simulink model "nl_cart_3"  (R2022a)
settings: Solver=ode45  StartTime=0.0  StopTime=40  MaxStep=0.001  MinStep=0.000001  RelTol=1e-3
values from neighbouring files (symbols this model uses):
  b = 0    [ex1.m]    (also in ex2.m = 1; ex3.m = 1; lab3es2_20230414.m = 1)
  dth0 = 0    [ex1.m]    (also in ex2.m; ex3.m)
  dx0 = 0    [ex1.m]    (also in ex2.m; ex3.m)
  g = 9.81    [ex1.m]    (also in ex2.m; ex3.m; lab3es2_20230414.m)
  Ie = I + m * l^2    (= 0.02603525)    [ex1.m]    (also in ex2.m; ex3.m; lab3es2_20230414.m = 0.026047)
  K = [k1, k2, k3, k4]    [ex3.m]    (also in lab3es2_20230414.m = [k,0,0,0])
  l = 0.305    [ex1.m]    (also in ex2.m; ex3.m; lab3es2_20230414.m)
  m = 0.21    [ex1.m]    (also in ex2.m; ex3.m; lab3es2_20230414.m)
  Me = M + m    (= 0.665)    [ex1.m]    (also in ex2.m; ex3.m; lab3es2_20230414.m)
  th0 = pi    (= 3.14159265359)    [ex1.m]    (also in ex2.m = 0; ex3.m = 0)
  x0 = 0    [ex1.m]    (also in ex2.m; ex3.m = 10)
undefined symbols (not defined in the file or in its folder): d
settings Model: Creator=loren  LastModifiedBy=loren
settings DataIOCC: ReturnWorkspaceOutputs=off

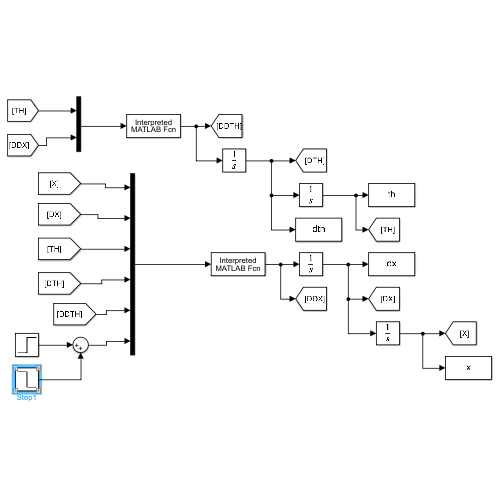
[thumbnail: Simulink's stored preview of the top-level diagram]
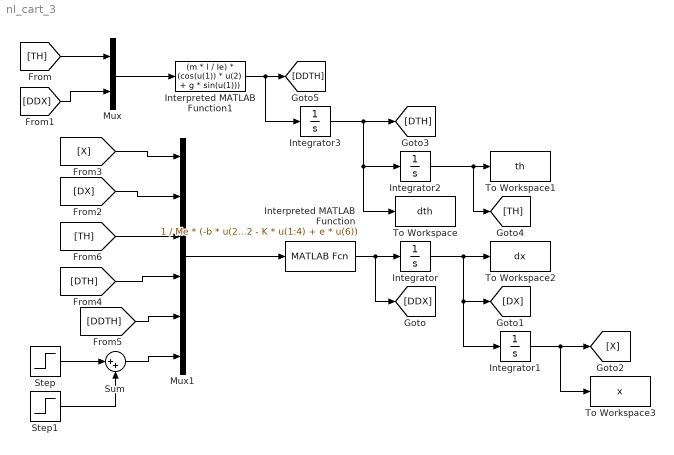
== system nl_cart_3 ==
  Integrator : Integrator  InitialCondition=dx0
  Integrator1 : Integrator  InitialCondition=x0
  Integrator2 : Integrator  InitialCondition=th0
  Integrator3 : Integrator  InitialCondition=dth0
  Interpreted MATLAB Function : MATLABFcn  MATLABFcn=1 / Me * (-b * u(2) + m * l * cos(u(3)) * u(5) - m * l * sin(u(3)) * u(4)^2 - K * u(1:4) + e * u(6))  OutputDimensions=1
  Interpreted MATLAB Function1 : MATLABFcn  MATLABFcn=(m * l / Ie) * (cos(u(1)) * u(2) + g * sin(u(1)))  OutputDimensions=1
  Mux : Mux  Inputs=2
  Mux1 : Mux  Inputs=6
  Step : Step  Time=d.start  After=d.A  SampleTime=0
  Step1 : Step  Time=d.end  After=-d.A  SampleTime=0
  Sum : Sum  Inputs=|++
  To Workspace : ToWorkspace  VariableName=dth  SaveFormat=Timeseries  SampleTime=-1
  To Workspace1 : ToWorkspace  VariableName=th  SaveFormat=Timeseries  SampleTime=-1
  To Workspace2 : ToWorkspace  VariableName=dx  SaveFormat=Timeseries  SampleTime=-1
  To Workspace3 : ToWorkspace  VariableName=x  SaveFormat=Timeseries  SampleTime=-1
  wires:
  Step1/1 -> Sum/2
  Mux/1 -> Interpreted MATLAB Function1/1
  Step/1 -> Sum/1
  Sum/1 -> Mux1/6
  [DTH] -> Mux1/4
  [TH] -> Mux/1
  [DX] -> Mux1/2
  [DDTH] -> Mux1/5
  Interpreted MATLAB Function1/1 -> [DDTH], Integrator3/1
  [X] -> Mux1/1
  Mux1/1 -> Interpreted MATLAB Function/1
  Integrator1/1 -> [X], To Workspace3/1
  [TH] -> Mux1/3
  Integrator2/1 -> [TH], To Workspace1/1
  Integrator/1 -> [DX], Integrator1/1, To Workspace2/1
  [DDX] -> Mux/2
  Integrator3/1 -> Integrator2/1, To Workspace/1, [DTH]
  Interpreted MATLAB Function/1 -> Integrator/1, [DDX]
